simulink model "ARI_26_1_Integrator_Nonlinear"  (Simulink 7.8)
settings: Solver=ode45  StartTime=0.0  StopTime=5  RelTol=1e-10
libraries: simulink x2
settings Model: Creator=Michael Sebek  ModifiedByFormat=Michael Sebek  LastModifiedBy=Michael Sebek
settings OptimizationCC: InitFltsAndDblsToZero=on
settings DebuggingCC: SaveWithParameterizedLinksMsg=none  SignalResolutionControl=TryResolveAllWithWarning  MultiTaskDSMMsg=warning  MultiTaskCondExecSysMsg=none  FcnCallInpInsideContextMsg=Use local settings  StrictBusMsg=None
settings RTWCC: IncludeERTFirstTime=on
settings GRTTargetCC: TargetFcnLib=ansi_tfl_tmw.mat

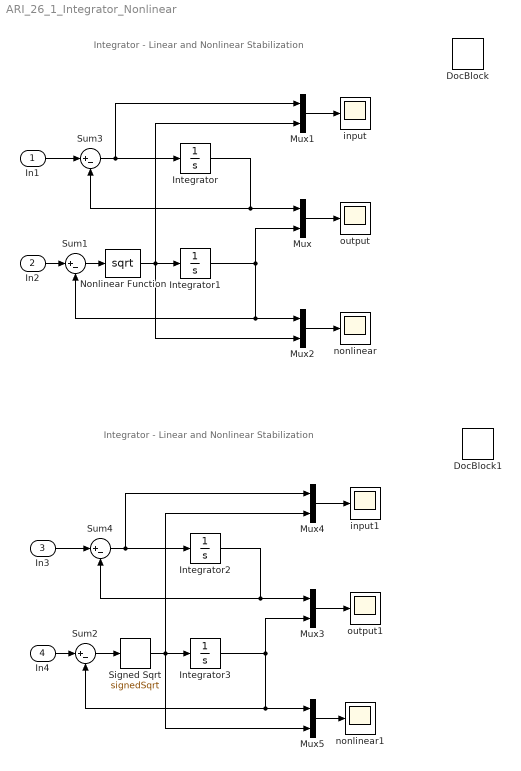
== system ARI_26_1_Integrator_Nonlinear ==
  note: Integrator - Linear and Nonlinear Stabilization
  note: Integrator - Linear and Nonlinear Stabilization
  In1 : Inport
  In2 : Inport  Port=2
  In3 : Inport  Port=3
  In4 : Inport  Port=4
  DocBlock : simulink/Model-Wide Utilities/DocBlock  DocumentType=Text
  DocBlock1 : simulink/Model-Wide Utilities/DocBlock  DocumentType=Text
  Integrator{,1..3} (4 alike) : Integrator  InitialCondition=1
  Mux{,1..5} (6 alike) : Mux  Inputs=2
  Nonlinear Function : Math  Operator=sqrt  OutputSignalType=real  SaturateOnIntegerOverflow=on
  Signed Sqrt : Sqrt  Operator=signedSqrt  SaturateOnIntegerOverflow=on
  Sum{1..4} (4 alike) : Sum  Inputs=|+-
  input : Scope
      settings: YMin=-1  YMax=0.05  SaveName=ScopeData2  MaxDataPoints=500000
  input1 : Scope
      settings: YMin=-1  YMax=0.05  MaxDataPoints=500000
  nonlinear : Scope
      settings: SaveName=ScopeData7  MaxDataPoints=500000
  nonlinear1 : Scope
      settings: MaxDataPoints=500000
  output : Scope
      settings: YMin=-8.67362e-019  YMax=0.01  SaveName=ScopeData3
  output1 : Scope
      settings: YMin=-8.67362e-019  YMax=0.01  SaveName=ScopeData4
  wires:
  Mux/1 -> output/1
  Mux1/1 -> input/1
  Sum3/1 -> Integrator/1, Mux1/1
  Integrator/1 -> Mux/1, Sum3/2
  Sum1/1 -> Nonlinear Function/1
  Integrator1/1 -> Mux2/1, Sum1/2, Mux/2
  Mux2/1 -> nonlinear/1
  In1/1 -> Sum3/1
  In2/1 -> Sum1/1
  Nonlinear Function/1 -> Integrator1/1, Mux1/2, Mux2/2
  Mux3/1 -> output1/1
  Mux4/1 -> input1/1
  Sum4/1 -> Integrator2/1, Mux4/1
  Integrator2/1 -> Mux3/1, Sum4/2
  Sum2/1 -> Signed Sqrt/1
  Integrator3/1 -> Mux5/1, Sum2/2, Mux3/2
  Mux5/1 -> nonlinear1/1
  In3/1 -> Sum4/1
  In4/1 -> Sum2/1
  Signed Sqrt/1 -> Integrator3/1, Mux4/2, Mux5/2
